simulink model "LPV_Demonstrator"  (R2018a)
settings: Solver=FixedStepAuto  StartTime=0.0  StopTime=FA.TMax  FixedStep=FA.DT  RelTol=1e-3  EnableMultiTasking=on
undefined symbols (not defined in the file or in its folder): Control, DiscIntNeverNeededParam, FA, k_opt, OutList, Parameters, PitchControlParams, rpm2radps, S_ConstTq, S_LowBPLim, strmatch, TorqueControlParams
libraries: simulink_extras x1
settings Model: ExtModeTrigMode=oneshot  ExtModeArmWhenConnect=off  Creator=Dana Martin  LastModifiedBy=dmartin
settings DataIOCC: SaveFormat=Array  SaveOutput=off  InspectSignalLogs=on  SignalLoggingName=sigsOut  OutputTimes=[0:500]/50
settings OptimizationCC: BooleanDataType=off  ExpressionDepthLimit=2147483647  InitFltsAndDblsToZero=on  LifeSpan=inf
settings DebuggingCC: SignalRangeChecking=warning  AlgebraicLoopMsg=error  SaveWithParameterizedLinksMsg=none  UnderspecifiedInitializationDetection=Classic  MergeDetectMultiDrivingBlocksExec=none  SignalResolutionControl=TryResolveAllWithWarning  TimeAdjustmentMsg=warning  MultiTaskDSMMsg=warning  MultiTaskCondExecSysMsg=warning  ParameterUnderflowMsg=warning  UnderSpecifiedDataTypeMsg=warning  UnnecessaryDatatypeConvMsg=warning  VectorMatrixConversionMsg=warning  FcnCallInpInsideContextMsg=warning  SignalLabelMismatchMsg=warning  SFcnCompatibilityMsg=warning  UniqueDataStoreMsg=warning  AllowSymbolicDim=off  ModelReferenceIOMsg=warning  ModelReferenceVersionMismatchMessage=warning  ModelReferenceIOMismatchMessage=warning  StateNameClashWarn=warning  StrictBusMsg=WarnOnBusTreatedAsVector  NonBusSignalsTreatedAsBus=warning  SFUnexpectedBacktrackingDiag=warning  SFNoUnconditionalDefaultTransitionDiag=warning  SFExecutionAtInitializationDiag=none
settings HardwareCC: ProdBitPerPointer=32  ProdBitPerSizeT=32  ProdBitPerPtrDiffT=32  ProdLargestAtomicFloat=None  ProdIntDivRoundTo=Undefined  ProdEndianess=Unspecified  ProdWordSize=32  ProdHWDeviceType=32-bit Generic  TargetBitPerPointer=64  TargetBitPerSizeT=64  TargetBitPerPtrDiffT=64  TargetLongLongMode=on  TargetIntDivRoundTo=Zero  TargetEndianess=LittleEndian  TargetWordSize=64  TargetHWDeviceType=MATLAB Host  ProdEqTarget=off
settings ModelReferenceCC: PropagateSignalLabelsOutOfModel=off
settings CodeAppCC: StateflowObjectComments=on
settings GRTTargetCC: TargetFcnLib=ansi_tfl_tmw.mat  TargetLangStandard=C89/C90 (ANSI)  ModelReferenceCompliant=off  GeneratePreprocessorConditionals=Disable all  CombineOutputUpdateFcns=off  GRTInterface=on
settings ConfigComp: CovMetricSettings=dw  CovHtmlReporting=on  CovSaveCumulativeToWorkspaceVar=on  CovSaveSingleToWorkspaceVar=on  CovExternalEMLEnable=off  CovSFcnEnable=off

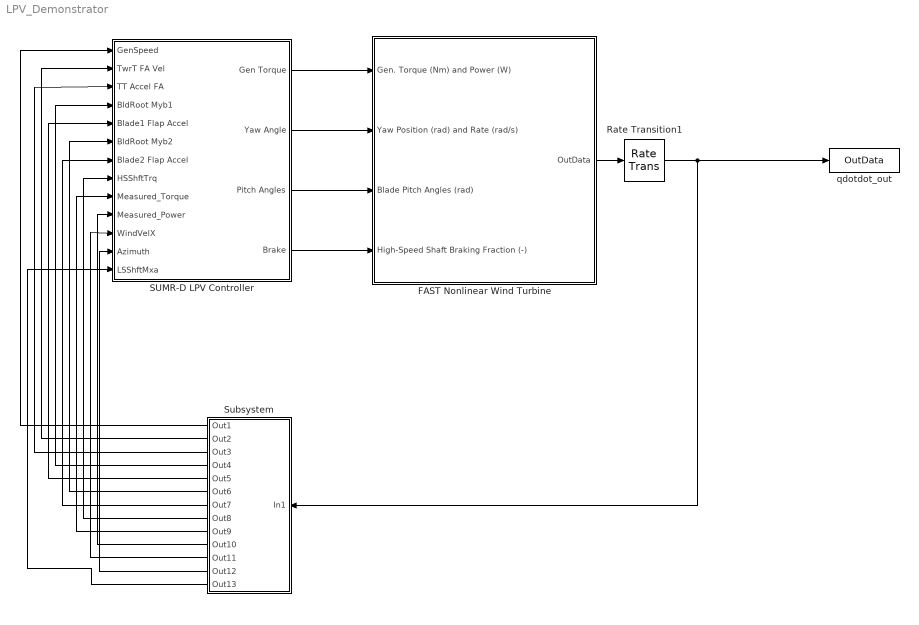
== system LPV_Demonstrator ==
  FAST Nonlinear Wind Turbine : Subsystem  mask(FAST Nonlinear Wind Turbine){}
      mask help: This block contains the FAST S-Function.
      mask init:
      | clear FAST_SFunc
  Rate Transition1 : RateTransition
  SUMR-D LPV Controller : Subsystem
  Subsystem : Subsystem
  qdotdot_out : ToWorkspace  VariableName=OutData  SaveFormat=Structure With Time  SampleTime=-1
  wires:
  SUMR-D LPV Controller/1(Gen Torque) -> FAST Nonlinear Wind Turbine/1(Gen. Torque (Nm) and Power (W))
  SUMR-D LPV Controller/3(Pitch Angles) -> FAST Nonlinear Wind Turbine/3(Blade Pitch Angles (rad))
  SUMR-D LPV Controller/2(Yaw Angle) -> FAST Nonlinear Wind Turbine/2(Yaw Position (rad) and Rate (rad/s))
  SUMR-D LPV Controller/4(Brake) -> FAST Nonlinear Wind Turbine/4(High-Speed Shaft Braking Fraction (-))
  Rate Transition1/1 -> Subsystem/1(In1), qdotdot_out/1
  FAST Nonlinear Wind Turbine/1(OutData) -> Rate Transition1/1
  Subsystem/1(Out1) -> SUMR-D LPV Controller/1(GenSpeed)
  Subsystem/2(Out2) -> SUMR-D LPV Controller/2(TwrT FA Vel)
  Subsystem/3(Out3) -> SUMR-D LPV Controller/3(TT Accel FA)
  Subsystem/4(Out4) -> SUMR-D LPV Controller/4(BldRoot Myb1)
  Subsystem/5(Out5) -> SUMR-D LPV Controller/5(Blade1 Flap Accel)
  Subsystem/6(Out6) -> SUMR-D LPV Controller/6(BldRoot Myb2)
  Subsystem/7(Out7) -> SUMR-D LPV Controller/7(Blade2 Flap Accel)
  Subsystem/8(Out8) -> SUMR-D LPV Controller/8(HSShftTrq)
  Subsystem/9(Out9) -> SUMR-D LPV Controller/9(Measured_Torque)
  Subsystem/10(Out10) -> SUMR-D LPV Controller/10(Measured_Power)
  Subsystem/11(Out11) -> SUMR-D LPV Controller/11(WindVelX)
  Subsystem/12(Out12) -> SUMR-D LPV Controller/12(Azimuth)
  Subsystem/13(Out13) -> SUMR-D LPV Controller/13(LSShftMxa)

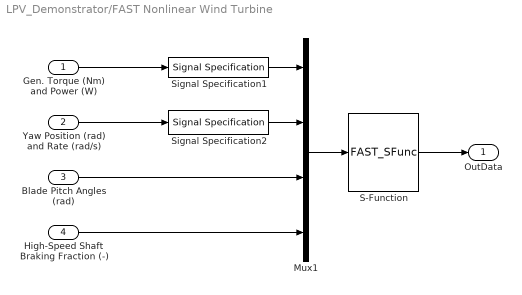
== system LPV_Demonstrator/FAST Nonlinear Wind Turbine ==
  Gen. Torque (Nm) and Power (W) : Inport
  Yaw Position (rad) and Rate (rad/s) : Inport  Port=2
  Blade Pitch Angles (rad) : Inport  Port=3
  High-Speed Shaft Braking Fraction (-) : Inport  Port=4
  Mux1 : Mux
  S-Function : S-Function  FunctionName=FAST_SFunc  Parameters=FAST_InputFileName, FA.TMax, 0  SFunctionDeploymentMode=off  EnableBusSupport=off
  Signal Specification1 : SignalSpecification  OutDataTypeStr=double  Dimensions=2
  Signal Specification2 : SignalSpecification  OutDataTypeStr=double  Dimensions=2
  OutData : Outport
  wires:
  Gen. Torque (Nm) and Power (W)/1 -> Signal Specification1/1
  S-Function/1 -> OutData/1
  Mux1/1 -> S-Function/1
  Blade Pitch Angles (rad)/1 -> Mux1/3
  Yaw Position (rad) and Rate (rad/s)/1 -> Signal Specification2/1
  Signal Specification1/1 -> Mux1/1
  Signal Specification2/1 -> Mux1/2
  High-Speed Shaft Braking Fraction (-)/1 -> Mux1/4

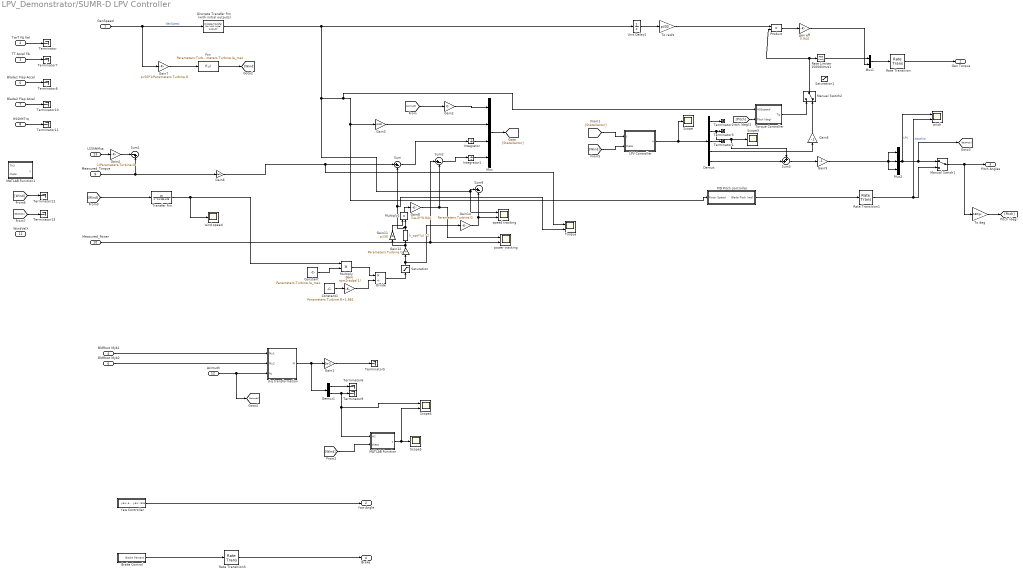
== system LPV_Demonstrator/SUMR-D LPV Controller ==
  GenSpeed : Inport
  TwrT FA Vel : Inport  Port=2
  TT Accel FA : Inport  Port=3
  BldRoot Myb1 : Inport  Port=4
  Blade1 Flap Accel : Inport  Port=5
  BldRoot Myb2 : Inport  Port=6
  Blade2 Flap Accel : Inport  Port=7
  HSShftTrq : Inport  Port=8
  Measured_Torque : Inport  Port=9
  Measured_Power : Inport  Port=10
  WindVelX : Inport  Port=11
  Azimuth : Inport  Port=12
  LSShftMxa : Inport  Port=13
  " " : Fcn  Expr=k_opt*(u)^2
  Brake Control : Subsystem
  Constant : Constant  Value=Parameters.Turbine.la_max  SampleTime=FA.DT
  Constant1 : Constant  Value=Parameters.Turbine.R+1.881
  Demux : Demux  Outputs=5
  Demux1 : Demux  Outputs=2
  Discrete Transfer Fcn (with initial outputs) : simulink_extras/Additional Discrete/Discrete Transfer Fcn (with initial outputs)  N=Parameters.LPF.LPnum  D=Parameters.LPF.LPden  U0=Parameters.Turbine.IC.Wg  Y0=Parameters.Turbine.IC.Wg  TS=FA.DT
      settings: SourceProductName=Simulink  SourceProductBaseCode=SL
  Divide : Product  Inputs=*/
  Fcn : Fcn  Expr=Parameters.Turbine.R*u(1)/Parameters.Turbine.la_max
  Gain : Gain  Gain=rpm2radps(1)
  Gain1 : Gain  Gain=1e-3
  Gain11 : Gain  Gain=pi/30
  Gain12 : Gain  Gain=Parameters.Turbine.G
  Gain14 : Gain  Gain=Parameters.Turbine.G
  Gain2 : Gain  Gain=0
  Gain3 : Gain  Gain=pi/30
  Gain4 : Gain  Gain=1/Parameters.Turbine.G
  Gain5 : Gain  Gain=-1
  Gain6 : Gain  Gain=1e3
  Gain7 : Gain  Gain=pi/30*1/Parameters.Turbine.G
  Gain8 : Gain  Gain=(1e-3)*0.944
  Gain9 : Gain  Gain=-1
  Integrator : Integrator
  Integrator1 : Integrator
  LPV Controller : Subsystem  TreatAsAtomicUnit=on
      settings: MinAlgLoopOccurrences=on
  MATLAB Function : MATLAB Function  TreatAsAtomicUnit=on
  MATLAB Function1 : MATLAB Function  TreatAsAtomicUnit=on
  Manual Switch1 : ManualSwitch
  Manual Switch2 : ManualSwitch  CurrentSetting=0
  Multiply : Product
  Multiply1 : Product
  Mux : Mux
  Mux1 : Mux  Inputs=2
  Mux2 : Mux  Inputs=3
  PID Pitch controller : Subsystem
      settings: MinAlgLoopOccurrences=on
  Product : Product  RndMeth=Zero
  Rate Limiter 15000Nm/s1 : RateLimiter  RisingSlewLimit=15000  FallingSlewLimit=-15000  SampleTimeMode=inherited
  Rate Transition : RateTransition  InitialCondition=Parameters.Turbine.IC.Tg
  Rate Transition1 : RateTransition  InitialCondition=Parameters.Turbine.IC.Tg
  Rate Transition3 : RateTransition
  Saturation : Saturate  UpperLimit=Parameters.Turbine.wr_rated  LowerLimit=0
  Saturation1 : Saturate  UpperLimit=Parameters.Turbine.T_rated  LowerLimit=0
  Scope : Scope
  Scope3 : Scope
  Scope4 : Scope  NumInputPorts=2
  Scope5 : Scope
  Sum : Sum  Inputs=|+-
  Sum1 : Sum  Inputs=|-+
  Sum2 : Sum  Inputs=|+-
  Sum3 : Sum  Inputs=++|
  Sum8 : Sum  Inputs=|+-
  Terminator{,1..3,5..13} (13 alike) : Terminator
  To deg : Gain  Gain=180/pi
  To rad/s : Gain  Gain=pi/30
  Torque : Scope  NumInputPorts=2
  Torque Controller : Subsystem
  Transfer Fcn : TransferFcn  Numerator=[25]  Denominator=[1 10 25]
  Unit Delay1 : UnitDelay  InitialCondition=Parameters.Turbine.IC.Wg  SampleTime=FA.DT
  Yaw Controller : Subsystem
  d-q transformation : MATLAB Function  TreatAsAtomicUnit=on
  gen eff : Gain  Gain=0.944
  pitch : Scope  NumInputPorts=2
  power tracking : Scope  NumInputPorts=2
  speed tracking : Scope  NumInputPorts=2
  wind speed : Scope
  Gen Torque : Outport
  Yaw Angle : Outport  Port=2
  Pitch Angles : Outport  Port=3
  Brake : Outport  Port=4
  wires:
  Mux1/1 -> Rate Transition/1
  Product/1 -> gen eff/1
  Unit Delay1/1 -> To rad/s/1
  To rad/s/1 -> Product/1
  gen eff/1 -> Mux1/2
  GenSpeed/1 -> Gain7/1, Discrete Transfer Fcn (with initial outputs)/1  "GenSpeed"
  Brake Control/1(Brake Percent) -> Rate Transition3/1
  Rate Transition3/1 -> Brake/1
  Yaw Controller/1(yaw and yaw rate) -> Yaw Angle/1
  Constant/1 -> Multiply/2
  Multiply/1 -> Divide/1
  Constant1/1 -> Gain/1
  Gain/1 -> Divide/2
  Azimuth/1 -> [Azimuth], d-q transformation/3(Az)
  LPV Controller/1(u) -> Scope/1, Demux/1
  Rate Transition/1 -> Gen Torque/1
  d-q transformation/1(M) -> Demux1/1, Gain1/1
  Gain1/1 -> Terminator5/1
  BldRoot Myb1/1 -> d-q transformation/1(My1)
  Multiply1/1 -> Gain8/1
  Gain11/1 -> Multiply1/1
  Divide/1 -> Saturation/1
  Gain12/1 -> Gain11/1, " "/1
  BldRoot Myb2/1 -> d-q transformation/2(My2)
  Rate Limiter 15000Nm/s1/1 -> Mux1/1
  [StateVector] -> LPV Controller/1(y)
  MATLAB Function/1(y) -> Scope4/2, Scope5/1
  Demux1/1 -> Terminator6/1
  Demux1/2 -> Scope4/1, MATLAB Function/1(H2), Terminator9/1
  [Wind] -> MATLAB Function/2(theta)
  Gain8/1 -> Sum2/2, power tracking/1
  [Wind] -> Transfer Fcn/1
  Demux/1 -> Terminator2/1
  Mux/1 -> [StateVector]
  [Pitch] -> Torque Controller/2(Pitch (deg))
  To deg/1 -> [Pitch]
  [Wind] -> LPV Controller/2(theta)
  Saturation/1 -> Gain12/1, Gain14/1
  Gain14/1 -> speed tracking/2, Sum8/2
  Mux2/1 -> pitch/1, Manual Switch1/1, [BldPitch]  "LPV"
  PID Pitch controller/1(Blade Pitch (rad)) -> Rate Transition1/1
  Rate Transition1/1 -> pitch/2, Manual Switch1/2  "baseline"
  Manual Switch1/1 -> Pitch Angles/1, To deg/1
  Measured_Power/1 -> Sum2/1, power tracking/2
  Gain6/1 -> Torque/1, Sum/1
  Measured_Torque/1 -> Sum1/2, Gain6/1
  LSShftMxa/1 -> Gain4/1
  Gain4/1 -> Sum1/1
  TwrT FA Vel/1 -> Terminator/1
  TT Accel FA/1 -> Terminator7/1
  Blade1 Flap Accel/1 -> Terminator8/1
  Blade2 Flap Accel/1 -> Terminator10/1
  HSShftTrq/1 -> Terminator11/1
  [Wind] -> Terminator12/1
  [BldPitch] -> Terminator13/1
  Torque Controller/1(Tg) -> Manual Switch2/1
  Integrator1/1 -> Mux/4
  [Azimuth] -> Gain2/1
  Gain2/1 -> Mux/1
  Discrete Transfer Fcn (with initial outputs)/1 -> Torque Controller/1(HSSspeed), Gain3/1, PID Pitch controller/1(Rotor Speed), speed tracking/1, Sum8/1, Unit Delay1/1
  Integrator/1 -> Mux/3
  " "/1 -> Torque/2, Sum/2, Multiply1/2
  Demux/3 -> Terminator1/1
  Gain3/1 -> Mux/2
  Demux/2 -> Sum3/1, Scope3/1, Terminator3/1
  Demux/4 -> Gain5/1
  Manual Switch2/1 -> Rate Limiter 15000Nm/s1/1, Product/2
  Transfer Fcn/1 -> wind speed/1, Multiply/1
  Gain7/1 -> Fcn/1
  Fcn/1 -> [Wind]
  Sum/1 -> Integrator/1
  Sum2/1 -> Integrator1/1
  Gain5/1 -> Manual Switch2/2
  Sum3/1 -> Gain9/1
  Demux/5 -> Sum3/2
  Gain9/1 -> Mux2/3, Mux2/1, Mux2/2

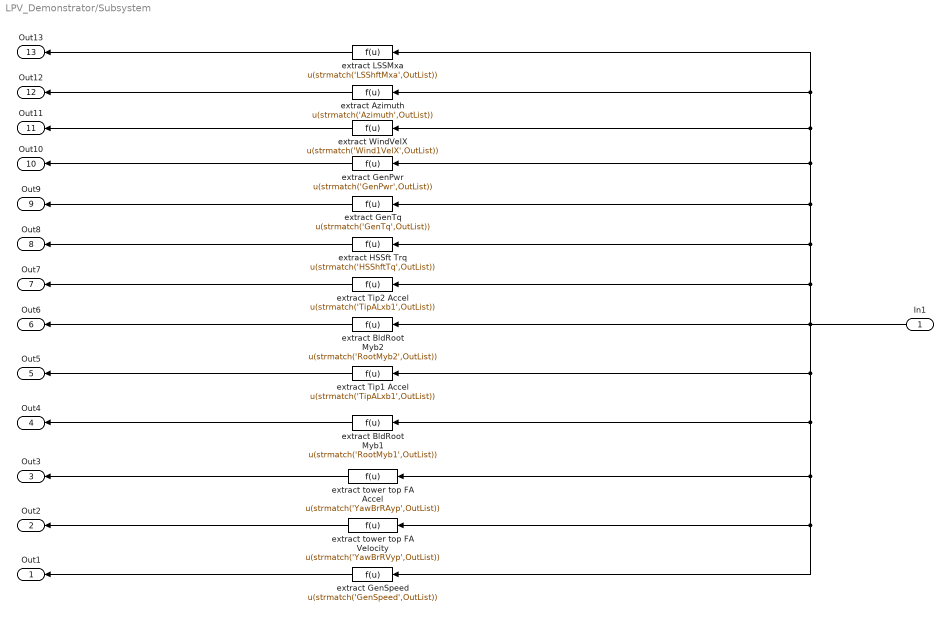
== system LPV_Demonstrator/Subsystem ==
  In1 : Inport
  extract Azimuth : Fcn  Expr=u(strmatch('Azimuth',OutList))
  extract BldRoot Myb1 : Fcn  Expr=u(strmatch('RootMyb1',OutList))
  extract BldRoot Myb2 : Fcn  Expr=u(strmatch('RootMyb2',OutList))
  extract GenPwr : Fcn  Expr=u(strmatch('GenPwr',OutList))
  extract GenSpeed : Fcn  Expr=u(strmatch('GenSpeed',OutList))
  extract GenTq : Fcn  Expr=u(strmatch('GenTq',OutList))
  extract HSSft Trq : Fcn  Expr=u(strmatch('HSShftTq',OutList))
  extract LSSMxa : Fcn  Expr=u(strmatch('LSShftMxa',OutList))
  extract Tip1 Accel : Fcn  Expr=u(strmatch('TipALxb1',OutList))
  extract Tip2 Accel : Fcn  Expr=u(strmatch('TipALxb1',OutList))
  extract WindVelX : Fcn  Expr=u(strmatch('Wind1VelX',OutList))
  extract tower top FA Accel : Fcn  Expr=u(strmatch('YawBrRAyp',OutList))
  extract tower top FA Velocity : Fcn  Expr=u(strmatch('YawBrRVyp',OutList))
  Out1 : Outport
  Out2 : Outport  Port=2
  Out3 : Outport  Port=3
  Out4 : Outport  Port=4
  Out5 : Outport  Port=5
  Out6 : Outport  Port=6
  Out7 : Outport  Port=7
  Out8 : Outport  Port=8
  Out9 : Outport  Port=9
  Out10 : Outport  Port=10
  Out11 : Outport  Port=11
  Out12 : Outport  Port=12
  Out13 : Outport  Port=13
  wires:
  extract WindVelX/1 -> Out11/1
  extract GenTq/1 -> Out9/1
  In1/1 -> extract LSSMxa/1, extract Azimuth/1, extract WindVelX/1, extract GenPwr/1, extract GenTq/1, extract HSSft Trq/1, extract Tip2 Accel/1, extract BldRoot Myb2/1, extract Tip1 Accel/1, extract BldRoot Myb1/1, extract tower top FA Velocity/1, extract GenSpeed/1, extract tower top FA Accel/1
  extract GenPwr/1 -> Out10/1
  extract Tip1 Accel/1 -> Out5/1
  extract HSSft Trq/1 -> Out8/1
  extract tower top FA Velocity/1 -> Out2/1
  extract tower top FA Accel/1 -> Out3/1
  extract Tip2 Accel/1 -> Out7/1
  extract Azimuth/1 -> Out12/1
  extract BldRoot Myb2/1 -> Out6/1
  extract GenSpeed/1 -> Out1/1
  extract BldRoot Myb1/1 -> Out4/1
  extract LSSMxa/1 -> Out13/1

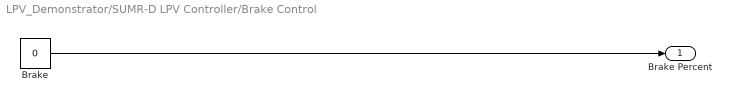
== system LPV_Demonstrator/SUMR-D LPV Controller/Brake Control ==
  Brake : Constant  Value=0  SampleTime=-1
  Brake Percent : Outport
  wires:
  Brake/1 -> Brake Percent/1

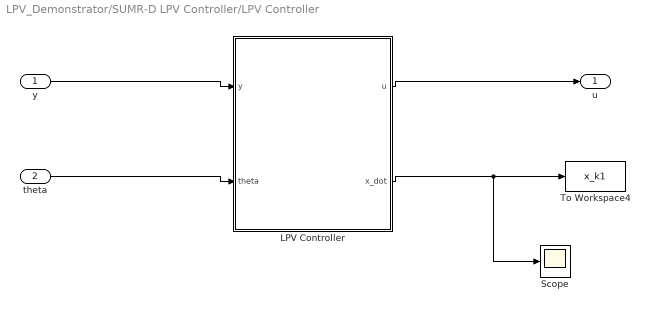
== system LPV_Demonstrator/SUMR-D LPV Controller/LPV Controller ==
  y : Inport
  theta : Inport  Port=2
  LPV Controller : MATLAB Function  TreatAsAtomicUnit=on  SystemSampleTime=FA.DT
      settings: MinAlgLoopOccurrences=on
  Scope : Scope
  To Workspace4 : ToWorkspace  VariableName=x_k1  SaveFormat=Structure With Time  SampleTime=-1
      settings: Decimation=3
  u : Outport
  wires:
  theta/1 -> LPV Controller/2(theta)
  y/1 -> LPV Controller/1(y)
  LPV Controller/1(u) -> u/1
  LPV Controller/2(x_dot) -> Scope/1, To Workspace4/1

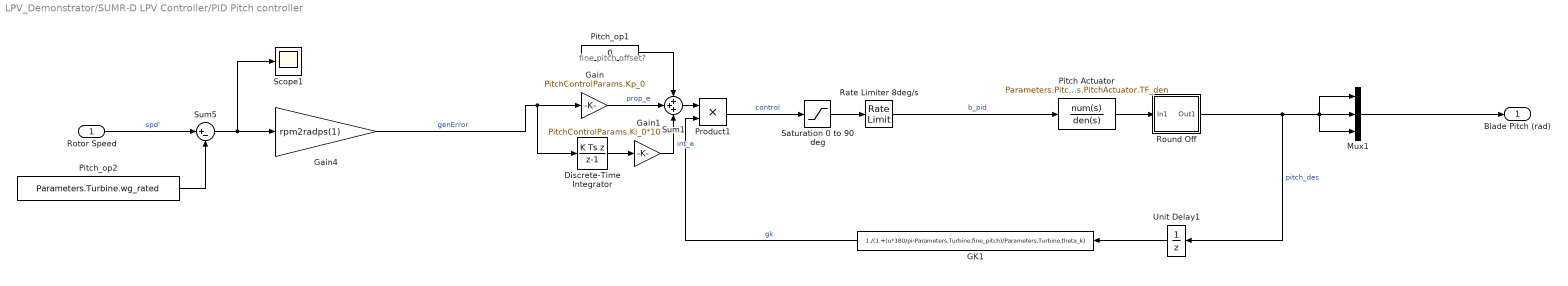
== system LPV_Demonstrator/SUMR-D LPV Controller/PID Pitch controller ==
  note: fine pitch offset?
  Rotor Speed : Inport
  Discrete-Time Integrator : DiscreteIntegrator  IntegratorMethod=Integration: Backward Euler  gainval=1  InitialCondition=deg2rad(Parameters.Turbine.fine_pitch)/(PitchControlParams.Ki_0)/(1./(1.+deg2rad(Parameters.Turbine.fine_pitch)/PitchControlParams.theta_k))  SampleTime=Control.DT  LimitOutput=on  UpperSaturationLimit=5*1.570796/(PitchControlParams.Ki_0)/(1./(1.+1.570796/PitchControlParams.theta_k))  LowerSaturationLimit=deg2rad(Parameters.Turbine.fine_pitch)/(PitchControlParams.Ki_0)/(1./(1.+deg2rad(Parameters.Turbine.fine_pitch)/PitchControlParams.theta_k))  ICPrevOutput=DiscIntNeverNeededParam  ICPrevScaledInput=DiscIntNeverNeededParam
  GK1 : Fcn  Expr=1./(1.+(u*180/pi-Parameters.Turbine.fine_pitch)/Parameters.Turbine.theta_k)
  Gain : Gain  Gain=PitchControlParams.Kp_0
  Gain1 : Gain  Gain=PitchControlParams.Ki_0*10
  Gain4 : Gain  Gain=rpm2radps(1)
  Mux1 : Mux  Inputs=3
  Pitch Actuator : TransferFcn  Numerator=Parameters.PitchActuator.TF_num  Denominator=Parameters.PitchActuator.TF_den
  Pitch_op1 : Constant  Value=0  SampleTime=Control.DT
  Pitch_op2 : Constant  Value=Parameters.Turbine.wg_rated  SampleTime=Control.DT
  Product1 : Product  RndMeth=Zero
  Rate Limiter 8deg/s : RateLimiter  RisingSlewLimit=18*pi/180  FallingSlewLimit=-18*pi/180  SampleTimeMode=inherited  InitialCondition=deg2rad(0)
  Round Off : Subsystem
  Saturation 0 to 90 deg : Saturate  UpperLimit=90*pi/180  LowerLimit=deg2rad(Parameters.Turbine.fine_pitch)
  Scope1 : Scope
  Sum1 : Sum  Inputs=+++
  Sum5 : Sum  Inputs=|+-  SaturateOnIntegerOverflow=on  InputSameDT=on  OutDataTypeStr=Inherit: Same as first input
  Unit Delay1 : UnitDelay  InitialCondition=Parameters.Turbine.IC.Wg  SampleTime=Control.DT
  Blade Pitch (rad) : Outport
  wires:
  Pitch_op2/1 -> Sum5/2
  Rotor Speed/1 -> Sum5/1  "spd'"
  Discrete-Time Integrator/1 -> Gain1/1
  Pitch_op1/1 -> Sum1/1
  Gain1/1 -> Sum1/3  "int_e"
  Sum1/1 -> Product1/1
  Saturation 0 to 90 deg/1 -> Rate Limiter 8deg/s/1
  Rate Limiter 8deg/s/1 -> Pitch Actuator/1  "b_pid"
  Sum5/1 -> Scope1/1, Gain4/1
  Round Off/1(Out1) -> Unit Delay1/1, Mux1/1, Mux1/3, Mux1/2  "pitch_des"
  Product1/1 -> Saturation 0 to 90 deg/1  "control"
  Gain4/1 -> Discrete-Time Integrator/1, Gain/1  "genError"
  Mux1/1 -> Blade Pitch (rad)/1
  Pitch Actuator/1 -> Round Off/1(In1)
  GK1/1 -> Product1/2  "gk"
  Unit Delay1/1 -> GK1/1
  Gain/1 -> Sum1/2  "prop_e"

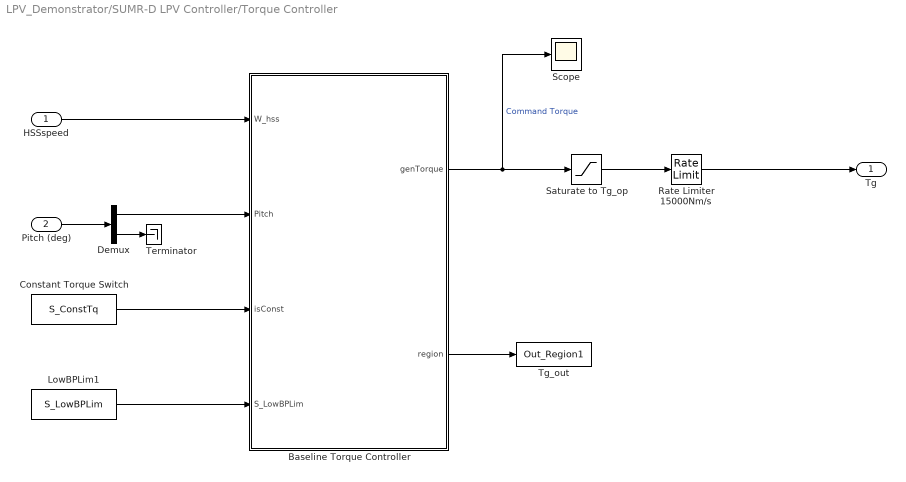
== system LPV_Demonstrator/SUMR-D LPV Controller/Torque Controller ==
  HSSspeed : Inport
  Pitch (deg) : Inport  Port=2
  Baseline Torque Controller : MATLAB Function  TreatAsAtomicUnit=on
  Constant Torque Switch : Constant  Value=S_ConstTq  SampleTime=Control.DT
  Demux : Demux  Outputs=[1, 2]
  LowBPLim1 : Constant  Value=S_LowBPLim  SampleTime=Control.DT
  Rate Limiter 15000Nm/s : RateLimiter  RisingSlewLimit=15000  FallingSlewLimit=-15000  SampleTimeMode=inherited
  Saturate to Tg_op : Saturate  UpperLimit=TorqueControlParams.T_rated  LowerLimit=0
  Scope : Scope
  Terminator : Terminator
  Tg_out : ToWorkspace  VariableName=Out_Region1  SampleTime=-1
      settings: MaxDataPoints=Inf
  Tg : Outport
  wires:
  Pitch (deg)/1 -> Demux/1
  Demux/2 -> Terminator/1
  Saturate to Tg_op/1 -> Rate Limiter 15000Nm/s/1
  Rate Limiter 15000Nm/s/1 -> Tg/1
  Baseline Torque Controller/1(genTorque) -> Saturate to Tg_op/1, Scope/1  "Command Torque"
  Baseline Torque Controller/2(region) -> Tg_out/1
  HSSspeed/1 -> Baseline Torque Controller/1(W_hss)
  Constant Torque Switch/1 -> Baseline Torque Controller/3(isConst)
  LowBPLim1/1 -> Baseline Torque Controller/4(S_LowBPLim)
  Demux/1 -> Baseline Torque Controller/2(Pitch)

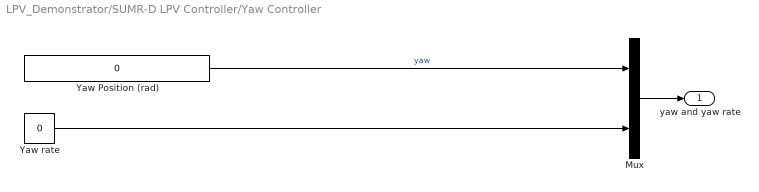
== system LPV_Demonstrator/SUMR-D LPV Controller/Yaw Controller ==
  Mux : Mux  Inputs=2
  Yaw Position (rad) : Constant  Value=0  SampleTime=-1
  Yaw rate : Constant  Value=0  SampleTime=-1
  yaw and yaw rate : Outport
  wires:
  Mux/1 -> yaw and yaw rate/1
  Yaw Position (rad)/1 -> Mux/1  "yaw"
  Yaw rate/1 -> Mux/2

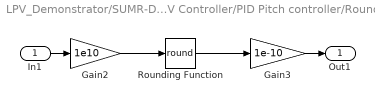
== system LPV_Demonstrator/SUMR-D LPV Controller/PID Pitch controller/Round Off ==
  In1 : Inport
  Gain2 : Gain  Gain=1e10
  Gain3 : Gain  Gain=1e-10
  Rounding Function : Rounding  Operator=round
  Out1 : Outport
  wires:
  Gain2/1 -> Rounding Function/1
  Rounding Function/1 -> Gain3/1
  Gain3/1 -> Out1/1
  In1/1 -> Gain2/1

== matlab function LPV_Demonstrator/SUMR-D LPV Controller/LPV Controller/LPV Controller ==
  data: y input; u output; x_dot output; theta input
function [u, x_dot]   = LPVController(y, theta)
coder.extrinsic('getGain');
persistent x_k

if isempty(x_k)
    x_k = zeros(3,1); 
end

K_bar       = zeros(8,8);
[K_bar]   = getGain_Gen(theta);

S.S1 = 1e-5;                                                                                   
S.S2 = 1e-5;

A_k        = S.S1*K_bar(1:3,1:3);
B_k        = S.S2*K_bar(1:3,5:8);
C_k        = S.S1*K_bar(4:8,1:3);
D_k        = S.S2*K_bar(4:8,5:8);

x_dot      = A_k*x_k+B_k*y;
u          = C_k*x_dot+D_k*y; 

x_k        = x_dot;
end

== matlab function LPV_Demonstrator/SUMR-D LPV Controller/MATLAB Function ==
  data: H2 input; y output; theta input
function y = fcn(H2,theta)

blade_bend = -0.0861*theta^2+1.7617*theta+11.9821;

y = H2-blade_bend;

end

== matlab function LPV_Demonstrator/SUMR-D LPV Controller/Torque Controller/Baseline Torque Controller ==
  settings: updateMethod=DISCRETE  sampleTime=Control.DT
  data: W_hss input; Pitch input; genTorque output; isConst input; region output; S_LowBPLim input; TorqueControlParams parameter
function [genTorque, region] = regionSelectTq_Flex( W_hss, Pitch, isConst, S_LowBPLim, TorqueControlParams)
% This block supports an embeddable subset of the MATLAB language.
% See the help menu for details.


%% Assign Constants

wg_rated    = TorqueControlParams.wg_rated;
T_rated     = TorqueControlParams.T_rated;
w2_high     = TorqueControlParams.w2_high;
w1_high     = TorqueControlParams.w1_high;
wg_min      = TorqueControlParams.wg_min;
m2_5        = TorqueControlParams.m2_5;
c2_5        = TorqueControlParams.c2_5;
m1_5        = TorqueControlParams.m1_5;
c1_5        = TorqueControlParams.c1_5;
k_opt       = TorqueControlParams.k_opt;
P0          = TorqueControlParams.P0;
T2_high     = m2_5 * w2_high + c2_5;

%% Switch based on Gen. Speed

if (((S_LowBPLim==0)&&(W_hss >= wg_rated)) || ((S_LowBPLim==1)&&((Pitch >= TorqueControlParams.fine_pitch+1) || (W_hss >= wg_rated)))) %Region 3 calcs
    region=3;
    if (isConst)
        genTorque = T_rated;
    else
        genTorque = 30/pi * P0 / W_hss;
    end
elseif (W_hss >= w2_high)                %Region 2.5
    region=2.5;    
    genTorque = m2_5 * W_hss + c2_5;
    
elseif (W_hss >= w1_high)                    %Region 2
    region=2;
    genTorque = k_opt * W_hss^2;
elseif (W_hss > wg_min)                    %Region 1.5
    region=1.5;
    genTorque = m1_5 * W_hss + c1_5;
else                                    %Region 1
    region=1;
    genTorque = 0;
end

== matlab function LPV_Demonstrator/SUMR-D LPV Controller/MATLAB Function1 ==
  data: TH2 input; y output; theta input
function y = fcn(TH2,theta)

twr_bend = -0.4224*theta^2+9.1668*theta+75.8989;

y = TH2-twr_bend;

end

== matlab function LPV_Demonstrator/SUMR-D LPV Controller/d-q transformation ==
  data: My1 input; My2 input; M output; Az input
function M  = fcn(My1,My2, Az)
% This block supports the Embedded MATLAB subset.
% See the help menu for details. 

[M] = [1/2, 1/2;-1/2, 1/2]*[My1;My2];

end
